simulink model "emo_1wr4di4_task"  (Simulink 3.00)
libraries: logiclib x7, genlib x4, mathlib x4, analoglib x2, arclib x2, execlib x1, inoutlib x1

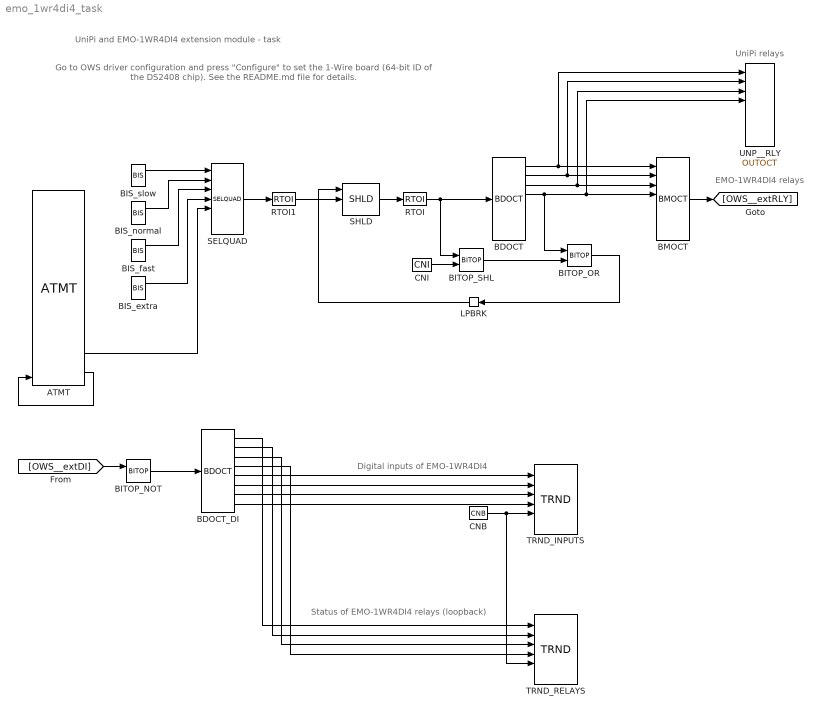
== system emo_1wr4di4_task ==
  note: UniPi relays
  note: EMO-1WR4DI4 relays
  note: Status of EMO-1WR4DI4 relays (loopback)
  note: Digital inputs of EMO-1WR4DI4
  note: Go to OWS driver configuration and press "Configure" to set the 1-Wire board (64-bit ID of the DS2408 chip).
      |
      | See the README.md file for details.
  note: UniPi and EMO-1WR4DI4 extension module - task
  ATMT : logiclib/ATMT  morestps=off  ntr=4  STT=[0 15 1; 1 15 2; 2 15 3; 3 15 0]  touts=[5.6 2.4 2.4 2.4 5 6 7 8 9 10 11 12 13 14 15 16]
  BDOCT : logiclib/BDOCT  shift=0
  BDOCT_DI : logiclib/BDOCT  shift=0
  BIS_extra : genlib/BIS  Y0=off  t1=0.05  t2=0.1  t3=0  t4=4  t5=5  t6=6  t7=7  t8=8  RPT=on
  BIS_fast : genlib/BIS  Y0=off  t1=0.1  t2=0.2  t3=0  t4=4  t5=5  t6=6  t7=7  t8=8  RPT=on
  BIS_normal : genlib/BIS  Y0=off  t1=0.2  t2=0.4  t3=0  t4=4  t5=5  t6=6  t7=7  t8=8  RPT=on
  BIS_slow : genlib/BIS  Y0=off  t1=0.4  t2=0.8  t3=0  t4=4  t5=5  t6=6  t7=7  t8=8  RPT=on
  BITOP_NOT : logiclib/BITOP  iop=1: Bit NOT
  BITOP_OR : logiclib/BITOP  iop=2: Bit OR
  BITOP_SHL : logiclib/BITOP  iop=5: Shift Left
  BMOCT : logiclib/BMOCT  shift=0
  CNB : mathlib/CNB  YCN=on
  CNI : mathlib/CNI  icn=1
  LPBRK : execlib/LPBRK  Orientation=left
  RTOI : mathlib/RTOI
  RTOI1 : mathlib/RTOI
  SELQUAD : analoglib/SELQUAD  BINF=off
  SHLD : analoglib/SHLD  y0=1  mode=1: Triggered sampling
  TRND_INPUTS : arclib/TRND  n=4  l=1000  btype=8: Double  ptype1=1: Store  ptype2=1: Store  ptype3=1: Store  ptype4=1: Store  pfac=1  afac=0  arc=0  id=1  Title=Status of the digital inputs  timesrc=1
  TRND_RELAYS : arclib/TRND  n=4  l=1000  btype=8: Double  ptype1=1: Store  ptype2=1: Store  ptype3=1: Store  ptype4=1: Store  pfac=1  afac=0  arc=0  id=1  Title=Status of the relays  timesrc=1
  UNP__RLY : inoutlib/OUTOCT
  wires:
  ATMT/17 -> SELQUAD/5
  ATMT/19 -> ATMT/20
  BDOCT/1 -> BMOCT/1, UNP__RLY/1
  BDOCT/2 -> BMOCT/2, UNP__RLY/2
  BDOCT/3 -> BMOCT/3, UNP__RLY/3
  BDOCT/4 -> BITOP_OR/1, BMOCT/4, UNP__RLY/4
  BDOCT_DI/1 -> TRND_RELAYS/1
  BDOCT_DI/2 -> TRND_RELAYS/2
  BDOCT_DI/3 -> TRND_RELAYS/3
  BDOCT_DI/4 -> TRND_RELAYS/4
  BDOCT_DI/5 -> TRND_INPUTS/1
  BDOCT_DI/6 -> TRND_INPUTS/2
  BDOCT_DI/7 -> TRND_INPUTS/3
  BDOCT_DI/8 -> TRND_INPUTS/4
  BIS_extra/1 -> SELQUAD/4
  BIS_fast/1 -> SELQUAD/3
  BIS_normal/1 -> SELQUAD/2
  BIS_slow/1 -> SELQUAD/1
  BITOP_NOT/1 -> BDOCT_DI/1
  BITOP_OR/1 -> LPBRK/1
  BITOP_SHL/1 -> BITOP_OR/2
  BMOCT/1 -> [OWS__extRLY]
  CNB/1 -> TRND_INPUTS/5, TRND_RELAYS/5
  CNI/1 -> BITOP_SHL/2
  [OWS__extDI] -> BITOP_NOT/1
  LPBRK/1 -> SHLD/1
  RTOI/1 -> BDOCT/1, BITOP_SHL/1
  RTOI1/1 -> SHLD/2
  SELQUAD/1 -> RTOI1/1
  SHLD/1 -> RTOI/1
